simulink model "Sun_Tracking_Solar_SystemV0"  (R2023a)
settings: Solver=VariableStepAuto  StartTime=0.0  StopTime=24*60*60  RelTol=1e-3
values from neighbouring files (symbols this model uses):
  J = 8.6    [VariablesAssigned.m]
  Kd = 5    [VariablesAssigned.m]
  Kf = 0.07    [VariablesAssigned.m]
  Kg = 2000    [VariablesAssigned.m]
  Kt = 10    [VariablesAssigned.m]
  L = 10    [VariablesAssigned.m]
  R = 500    [VariablesAssigned.m]
libraries: slpidlib x1
settings Model: Creator=M3tal  LastModifiedBy=M3tal
settings SolverCC: AlgebraicLoopSolver=TrustRegion
settings DataIOCC: ExternalInput=[sunTime, sunPosition]  LoadExternalInput=on
settings DebuggingCC: UnconnectedInputMsg=warning  UnconnectedOutputMsg=warning  UnconnectedLineMsg=warning  UnderSpecifiedDimensionMsg=warning
settings ModelReferenceCC: EnableRefExpFcnMdlSchedulingChecks=on

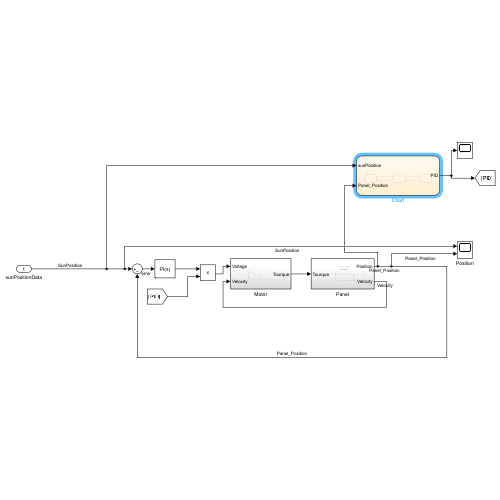
[thumbnail: Simulink's stored preview of the top-level diagram]
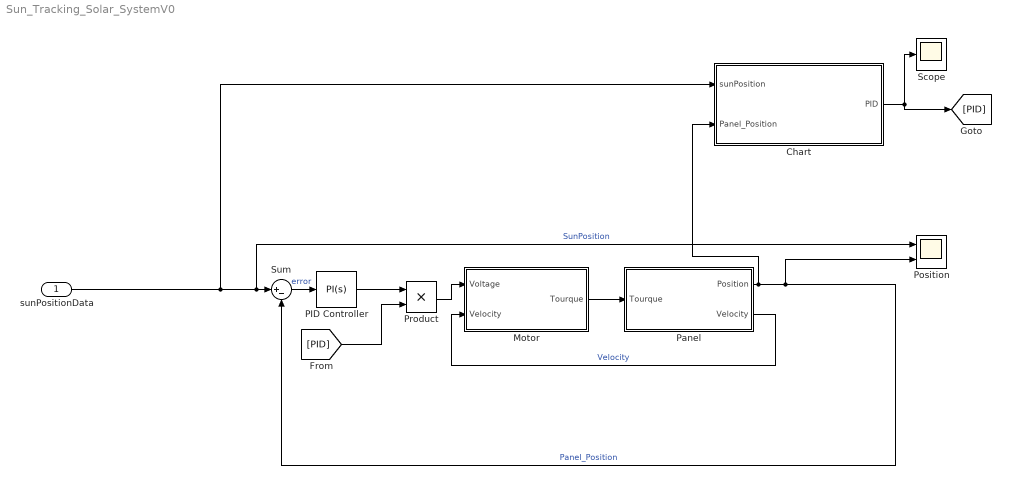
== system Sun_Tracking_Solar_SystemV0 ==
  sunPositionData : Inport
  Chart : Stateflow chart  TreatAsAtomicUnit=on
  Motor : Subsystem
  PID Controller : slpidlib/PID Controller  Controller=PI  Form=Parallel  TimeDomain=Continuous-time  UseExternalTs=off  SampleTime=-1  IntegratorMethod=Forward Euler  FilterMethod=Forward Euler  ControllerParametersSource=internal  P=180  I=100  UseKiTs=off  D=0  N=100  UseFilter=on  TunerSelectOption=Transfer Function Based (PID Tuner App)  InitialConditionSource=internal  InitialConditionForIntegrator=0  InitialConditionForFilter=0  DifferentiatorICPrevScaledInput=0  ExternalReset=none  TrackingMode=off  Kt=1  LimitOutput=off  SatLimitsSource=internal  UpperSaturationLimit=inf  LowerSaturationLimit=-inf  LinearizeAsGain=on  AntiWindupMode=none  Kb=1  LimitIntegrator=off  UpperIntegratorSaturationLimit=inf  LowerIntegratorSaturationLimit=-inf  POutMin=[]  POutMax=[]  IOutMin=[]  IOutMax=[]  DOutMin=[]  DOutMax=[]  NOutMin=[]  NOutMax=[]  SumOutMin=[]  SumOutMax=[]  SaturationOutMin=[]  SaturationOutMax=[]  PParamMin=[]  PParamMax=[]  IParamMin=[]  IParamMax=[]  DParamMin=[]  DParamMax=[]  NParamMin=[]  NParamMax=[]  KbParamMin=[]  KbParamMax=[]  KtParamMin=[]  KtParamMax=[]  KbOutMin=[]  KbOutMax=[]  KtOutMin=[]  KtOutMax=[]  IntegratorOutMin=[]  IntegratorOutMax=[]  FilterOutMin=[]  FilterOutMax=[]  SumI1OutMin=[]  SumI1OutMax=[]  SumI2OutMin=[]  SumI2OutMax=[]  SumI3OutMin=[]  SumI3OutMax=[]  SumI4OutMin=[]  SumI4OutMax=[]  SumDOutMin=[]  SumDOutMax=[]  DifferentiatorOutMin=[]  DifferentiatorOutMax=[]  FilterDiffOutCoefMin=[]  FilterDiffOutCoefMax=[]  ReciprocalOutMin=[]  ReciprocalOutMax=[]  SumDenOutMin=[]  SumDenOutMax=[]  SumNumOutMin=[]  SumNumOutMax=[]  DivideOutMin=[]  DivideOutMax=[]  UdiffTsProdOutMin=[]  UdiffTsProdOutMax=[]  NTsProdOutMin=[]  NTsProdOutMax=[]  UintegralTsProdOutMin=[]  UintegralTsProdOutMax=[]  UngainTsProdOutMin=[]  UngainTsProdOutMax=[]  ClampingZeroOutDataTypeStr=Inherit: Inherit via back propagation  ClampingZeroOutMin=[]  ClampingZeroOutMax=[]  FilterDenConstantOutDataTypeStr=Inherit: Inherit via back propagation  FilterDenConstantOutMin=[]  FilterDenConstantOutMax=[]  PCopyOutDataTypeStr=Inherit: Inherit via back propagation  PCopyOutMin=[]  PCopyOutMax=[]  NCopyOutDataTypeStr=Inherit: Inherit via back propagation  NCopyOutMin=[]  NCopyOutMax=[]  IntegratorContinuousStateAttributes=''  IntegratorStateMustResolveToSignalObject=off  IntegratorRTWStateStorageClass=Auto  FilterContinuousStateAttributes=''  FilterStateMustResolveToSignalObject=off  FilterRTWStateStorageClass=Auto  ParallelPVariant=InternalParameters  IdealPVariant=Disabled  IVariant=InternalParameters  DVariant=Disabled  IntegratorVariant=Continuous  SatVariant=Disabled  AWVariant=Passthrough  PCopyVariant=Disabled  TRVariant=Disabled  FdbkBlocksVariant=Forward  IdealPFdbkVariant=Disabled  SatFdbkVariant=Disabled  DerivativeFilterVariant=Disabled  NVariant=Disabled  NCopyVariant=Disabled_SignalSpec  FilterICVariant=Disabled  IntegratorICVariant=InternalICs  ExternalResetVariant=Disabled  TRSumVariant=Passthrough  SumFdbkVariant=Disabled  SumVariant=Sum_PI  TsampFilterVariant=InternalTs  TsampNgainVariant=Passthrough  TsampIntegralVariant=Disabled_SignalSpec  ExternalSaturationOutDataTypeStr=Inherit: Same as second input
  Panel : Subsystem
  Position : Scope  NumInputPorts=2
  Product : Product
  Scope : Scope
  Sum : Sum  Inputs=|+-
  wires:
  Motor/1(Tourque) -> Panel/1(Tourque)
  Panel/2(Velocity) -> Motor/2(Velocity)  "Velocity"
  sunPositionData/1 -> Chart/1(sunPosition), Position/1, Sum/1  "SunPosition"
  Sum/1 -> PID Controller/1  "error"
  PID Controller/1 -> Product/1
  Panel/1(Position) -> Chart/2(Panel_Position), Position/2, Sum/2  "Panel_Position"
  Chart/1(PID) -> [PID], Scope/1
  [PID] -> Product/2
  Product/1 -> Motor/1(Voltage)

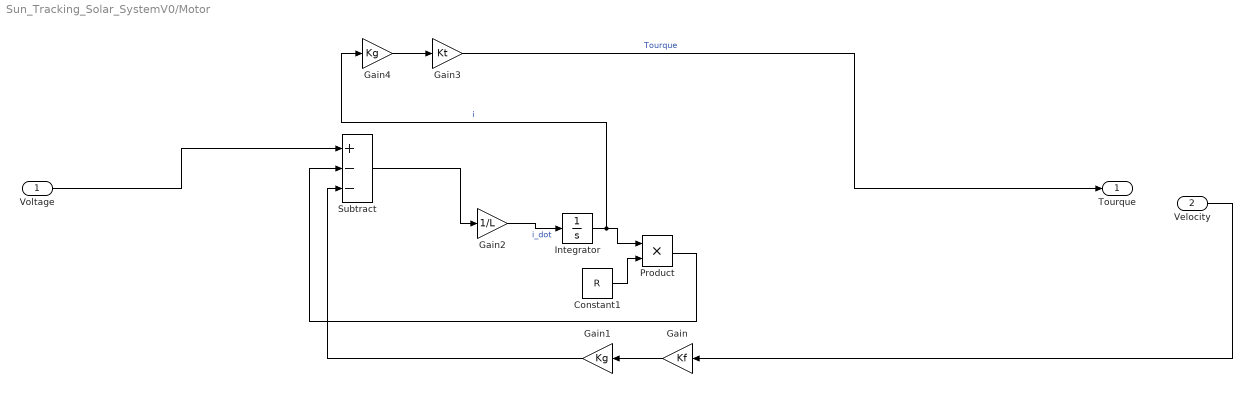
== system Sun_Tracking_Solar_SystemV0/Motor ==
  Voltage : Inport
  Velocity : Inport  Port=2
  Constant1 : Constant  Value=R
  Gain : Gain  Gain=Kf
  Gain1 : Gain  Gain=Kg
  Gain2 : Gain  Gain=1/L
  Gain3 : Gain  Gain=Kt
  Gain4 : Gain  Gain=Kg
  Integrator : Integrator
  Product : Product
  Subtract : Sum  Inputs=+--
  Tourque : Outport
  wires:
  Gain2/1 -> Integrator/1  "i_dot"
  Product/1 -> Subtract/2
  Subtract/1 -> Gain2/1
  Gain/1 -> Gain1/1
  Integrator/1 -> Product/1, Gain4/1  "i"
  Constant1/1 -> Product/2
  Velocity/1 -> Gain/1
  Gain1/1 -> Subtract/3
  Gain4/1 -> Gain3/1
  Gain3/1 -> Tourque/1  "Tourque"
  Voltage/1 -> Subtract/1

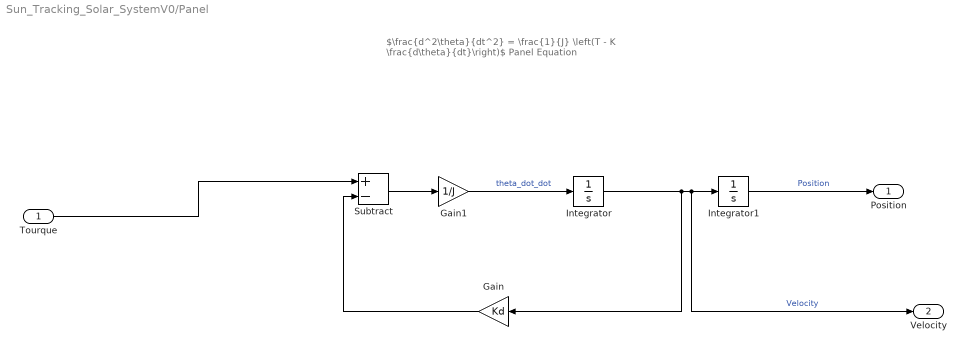
== system Sun_Tracking_Solar_SystemV0/Panel ==
  note: $\frac{d^2\theta}{dt^2} = \frac{1}{J} \left(T - K \frac{d\theta}{dt}\right)$
      | Panel Equation
  Tourque : Inport
  Gain : Gain  Gain=Kd
  Gain1 : Gain  Gain=1/J
  Integrator : Integrator
  Integrator1 : Integrator
  Subtract : Sum  Inputs=+-
  Position : Outport
  Velocity : Outport  Port=2
  wires:
  Gain/1 -> Subtract/2
  Integrator/1 -> Gain/1, Velocity/1, Integrator1/1  "Velocity"
  Tourque/1 -> Subtract/1
  Integrator1/1 -> Position/1  "Position"
  Gain1/1 -> Integrator/1  "theta_dot_dot"
  Subtract/1 -> Gain1/1

== stateflow chart Sun_Tracking_Solar_SystemV0/Chart ==
  state Tracking
    entry:
    PID=1
  state Stop
    entry:
    PID=0
  state Return
    entry:
    PID=-1
  (default) -> Tracking
  Tracking -> Stop : [Panel_Position==sunPosition(end)]
  Stop -> Return [order 1] : [PID==0]
  Stop -> Tracking [order 2] : [Panel_Position==sunPosition(1)&&PID==0]
  Return -> Stop : [Panel_Position==sunPosition(1)]
  data: sunPosition input; Panel_Position input; PID output
